simulink model "bipolar_unipolar_single_phase_inverter"  (R2018b)
settings: Solver=VariableStepDiscrete  StartTime=0.0  StopTime=0.1  RelTol=1e-3
libraries: powerlib x15, simulink x3
settings Model: Creator=verma  LastModifiedBy=verma

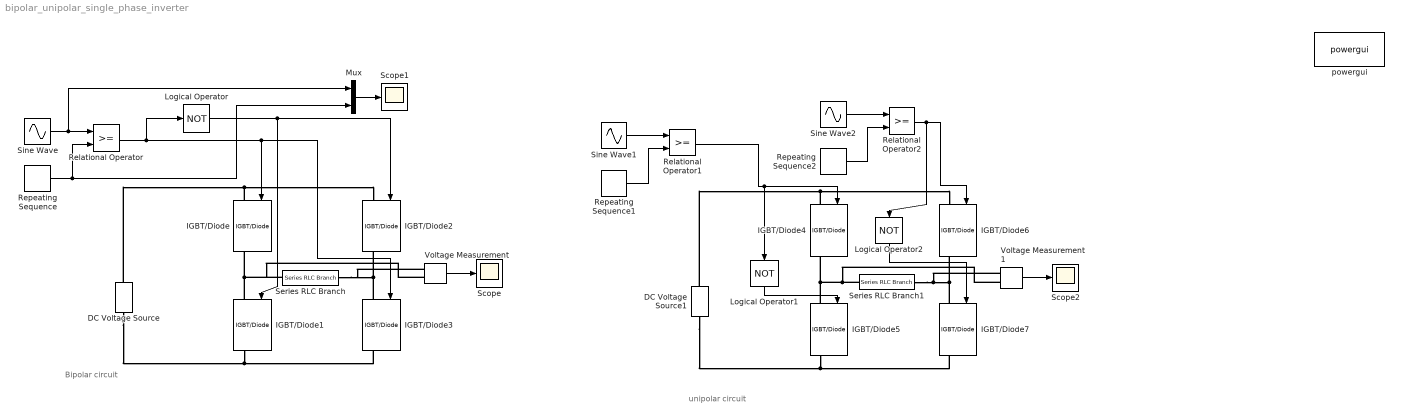
== system bipolar_unipolar_single_phase_inverter ==
  note: unipolar circuit
  note: Bipolar circuit
  DC Voltage Source : powerlib/Electrical Sources/DC Voltage Source  Amplitude=100  Measurements=None
  DC Voltage Source1 : powerlib/Electrical Sources/DC Voltage Source  Amplitude=100  Measurements=None
  IGBT/Diode{,1..7} (8 alike) : powerlib/Power Electronics/IGBT//Diode  Ron=1e-3  Rs=1e5  Cs=inf  Measurements=on
  Logical Operator : Logic  Operator=NOT  AllPortsSameDT=off  OutDataTypeStr=boolean
  Logical Operator1 : Logic  Operator=NOT  AllPortsSameDT=off  OutDataTypeStr=boolean
  Logical Operator2 : Logic  Operator=NOT  AllPortsSameDT=off  OutDataTypeStr=boolean
  Mux : Mux  Inputs=2
  Relational Operator : RelationalOperator  OutDataTypeStr=boolean  RndMeth=Simplest
  Relational Operator1 : RelationalOperator  OutDataTypeStr=boolean  RndMeth=Simplest
  Relational Operator2 : RelationalOperator  OutDataTypeStr=boolean  RndMeth=Simplest
  Repeating Sequence : simulink/Sources/Repeating Sequence  rep_seq_t=[0 (1/5050)/4 (1/5050)/2 (3/5050)/4 (1/5050)]  rep_seq_y=[0 1 0 -1 0]
  Repeating Sequence1 : simulink/Sources/Repeating Sequence  rep_seq_t=[0 (1/5050)/4 (1/5050)/2 (3/5050)/4 (1/5050)]  rep_seq_y=[0 1 0 -1 0]
  Repeating Sequence2 : simulink/Sources/Repeating Sequence  rep_seq_t=[0 (1/5050)/4 (1/5050)/2 (3/5050)/4 (1/5050)]  rep_seq_y=[0 1 0 -1 0]
  Scope : Scope
  Scope1 : Scope
  Scope2 : Scope
  Series RLC Branch : powerlib/Elements/Series RLC Branch  LConnTagsString=__new0  RConnTagsString=__new0  BranchType=R  Resistance=10  Inductance=1e-3  SetiL0=off  InitialCurrent=0  Capacitance=1e-6  Setx0=off  InitialVoltage=0  Measurements=None
  Series RLC Branch1 : powerlib/Elements/Series RLC Branch  LConnTagsString=__new0  RConnTagsString=__new0  BranchType=R  Resistance=10  Inductance=1e-3  SetiL0=off  InitialCurrent=0  Capacitance=1e-6  Setx0=off  InitialVoltage=0  Measurements=None
  Sine Wave : Sin  Amplitude=0.95  Frequency=2*pi*50  SampleTime=0
  Sine Wave1 : Sin  Amplitude=0.95  Frequency=2*pi*50  SampleTime=0
  Sine Wave2 : Sin  Amplitude=0.95  Frequency=2*pi*50  Phase=pi  SampleTime=0
  Voltage Measurement : powerlib/Measurements/Voltage Measurement  PhasorSimulation=off  OutputType=Complex  PSBequivalent=0
  Voltage Measurement1 : powerlib/Measurements/Voltage Measurement  PhasorSimulation=off  OutputType=Complex  PSBequivalent=0
  powergui : powerlib/powergui  Priority=1  SimulationMode=Discrete  SampleTime=1e-6  frequency=60  Iterations=50  frequencyindice=0  Pbase=100e6  ErrMax=1e-4  UnitsV=kV  UnitsW=MW  buscounter=0  FunctionMessages=off  echomessages=off  EnableUseOfTLC=off  CurrentSourceSwitches=off  DisableSnubberDevices=off  DisableRonSwitches=off  DisableVfSwitches=off  DisplayEquations=off  SolverType=Tustin/Backward Euler (TBE)  Interpol=off  ExternalGateDelay=off  methode=off  Ts=100  x0status=blocks  SPID=on  SwTol=0  HookPort=off  RestoreLinks=warning  ResistiveCurrentMeasurement=off  Frange=[0:2:500]  Ylog=off  Xlog=on  ShowGrid=off  save=off  variable=ZData  structure=v  ZoomFFT=off  StartTime=0.0  cycles=1  DisplayStyle=1  fundamental=50  FreqAxis=off  MaxFrequency=1000  frequencyindicesteady=1  RmsSteady=1  display=off
  wires:
  Voltage Measurement/1 -> Scope/1
  Sine Wave/1 -> Mux/1, Relational Operator/1
  Repeating Sequence/1 -> Mux/2, Relational Operator/2
  Relational Operator/1 -> Logical Operator/1, IGBT/Diode3/1, IGBT/Diode/1
  Logical Operator/1 -> IGBT/Diode2/1, IGBT/Diode1/1
  Mux/1 -> Scope1/1
  Voltage Measurement1/1 -> Scope2/1
  Sine Wave1/1 -> Relational Operator1/1
  Repeating Sequence1/1 -> Relational Operator1/2
  Sine Wave2/1 -> Relational Operator2/1
  Repeating Sequence2/1 -> Relational Operator2/2
  Relational Operator1/1 -> Logical Operator1/1, IGBT/Diode4/1
  Logical Operator1/1 -> IGBT/Diode5/1
  Relational Operator2/1 -> IGBT/Diode6/1, Logical Operator2/1
  Logical Operator2/1 -> IGBT/Diode7/1
  connections:
  IGBT/Diode/LConn1 -- IGBT/Diode2/LConn1 -- DC Voltage Source/RConn1
  IGBT/Diode1/RConn1 -- IGBT/Diode3/RConn1 -- DC Voltage Source/LConn1
  IGBT/Diode1/LConn1 -- Voltage Measurement/LConn2 -- Series RLC Branch/LConn1 -- IGBT/Diode/RConn1
  IGBT/Diode3/LConn1 -- Voltage Measurement/LConn1 -- Series RLC Branch/RConn1 -- IGBT/Diode2/RConn1
  Series RLC Branch1/RConn1 -- Voltage Measurement1/LConn1 -- IGBT/Diode6/RConn1 -- IGBT/Diode7/LConn1
  Series RLC Branch1/LConn1 -- Voltage Measurement1/LConn2 -- IGBT/Diode4/RConn1 -- IGBT/Diode5/LConn1
  IGBT/Diode5/RConn1 -- IGBT/Diode7/RConn1 -- DC Voltage Source1/LConn1
  IGBT/Diode4/LConn1 -- IGBT/Diode6/LConn1 -- DC Voltage Source1/RConn1
